simulink model "scout"  (R2018a)
settings: Solver=FixedStepDiscrete  StartTime=0.0  StopTime=300  FixedStep=0.1  RelTol=1e-3  EnableMultiTasking=on
libraries: simulink x1
settings Model: EnablePacing=on  PacingRate=0.180000  Creator=besho  LastModifiedBy=besho
settings SolverCC: AutoInsertRateTranBlk=on
settings DataIOCC: LimitDataPoints=on
settings OptimizationCC: LifeSpan=inf
settings DebuggingCC: AllowSymbolicDim=off  SFUnexpectedBacktrackingDiag=warning  SFNoUnconditionalDefaultTransitionDiag=warning  SFExecutionAtInitializationDiag=none
settings SFSimCC: SimCustomHeaderCode="#include \"main_scout.h\""  SimUserSources=main_scout.c
settings CodeAppCC: StateflowObjectComments=on
settings GRTTargetCC: TargetLangStandard=C89/C90 (ANSI)  GeneratePreprocessorConditionals=Disable all
settings ConfigComp: CovMetricSettings=dw  CovHtmlReporting=on  CovSaveCumulativeToWorkspaceVar=on  CovSaveSingleToWorkspaceVar=on  CovShowResultsExplorer=off  CovExternalEMLEnable=off  CovSFcnEnable=off

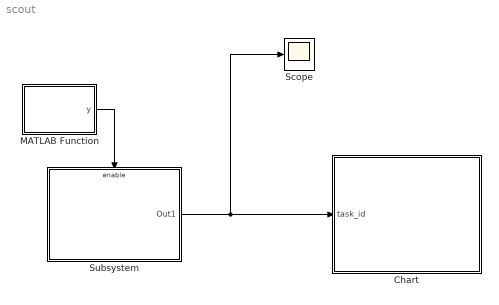
== system scout ==
  Chart : Stateflow chart  TreatAsAtomicUnit=on
  MATLAB Function : MATLAB Function  TreatAsAtomicUnit=on
  Scope : Scope
  Subsystem : Subsystem
  wires:
  MATLAB Function/1(y) -> Subsystem/Enable
  Subsystem/1(Out1) -> Scope/1, Chart/1(task_id)

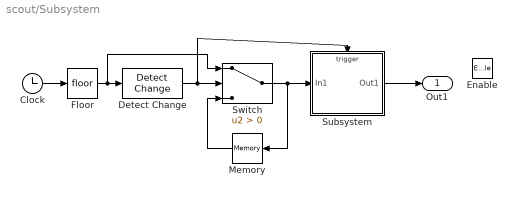
== system scout/Subsystem ==
  Enable : EnablePort  StatesWhenEnabling=reset
  Clock : Clock
  Detect Change : simulink/Logic and Bit Operations/Detect Change  vinit=0  OutDataTypeStr=boolean
  Floor : Rounding
  Memory : Memory
  Subsystem : Subsystem
  Switch : Switch  Criteria=u2 > Threshold
  Out1 : Outport
  wires:
  Clock/1 -> Floor/1
  Floor/1 -> Detect Change/1, Switch/1
  Detect Change/1 -> Switch/2, Subsystem/Trigger
  Switch/1 -> Subsystem/1(In1), Memory/1
  Memory/1 -> Switch/3
  Subsystem/1(Out1) -> Out1/1

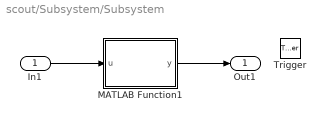
== system scout/Subsystem/Subsystem ==
  In1 : Inport
  Trigger : TriggerPort  VariantControl=Variant  PortDimensions=1
  MATLAB Function1 : MATLAB Function  TreatAsAtomicUnit=on
  Out1 : Outport
  wires:
  MATLAB Function1/1(y) -> Out1/1
  In1/1 -> MATLAB Function1/1(u)

== matlab function scout/Subsystem/Subsystem/MATLAB Function1 ==
  data: u input; y output
function y = sch_scout(u)
    y = 0;
    y = coder.ceval('schedule_scout_wrapper', u);
end

== matlab function scout/MATLAB Function ==
  data: y output
function y = init()
    y = 0;
    y = coder.ceval('init');
end

== stateflow chart scout/Chart ==
  state idle
  state sensor_sampling
  state rf_comms
  (default) -> idle
  idle -> sensor_sampling [order 1] : [task_id==1]
  sensor_sampling -> idle [order 2] : [task_id==5]
  idle -> rf_comms [order 2] : [task_id==2]
  rf_comms -> idle [order 1] : [task_id==5]
  rf_comms -> sensor_sampling [order 2] : [task_id==1]
  sensor_sampling -> rf_comms [order 1] : [task_id==2]
  data: task_id input
